simulink model "LQDG_Yaw"  (R2020a)
settings: Solver=ode3  StartTime=0.0  StopTime=10.0  FixedStep=0.01  RelTol=1e-3  EnableMultiTasking=on
undefined symbols (not defined in the file): weighting_matrix
libraries: arduinolib x5
settings Model: SILPILModeSetting=veronly  ExtModeTrigDuration=2  Creator=Ali  LastModifiedBy=Ali
settings OptimizationCC: EnhancedBackFolding=on  PassReuseOutputArgsAs=Individual arguments  ZeroExternalMemoryAtStartup=off  ZeroInternalMemoryAtStartup=off  MaxStackSize=64  OptimizeBlockOrder=speed  DifferentSizesBufferReuse=on  OptimizationCustomize=off  EfficientTunableParamExpr=on
settings DebuggingCC: ParameterTunabilityLossMsg=error
settings HardwareCC: ProdBitPerInt=16  ProdBitPerPointer=16  ProdBitPerSizeT=16  ProdBitPerPtrDiffT=16  ProdLargestAtomicFloat=None  ProdWordSize=8  ProdHWDeviceType=Atmel->AVR
settings SFSimCC: MATLABDynamicMemAlloc=off
settings RTWCC: SystemTargetFile=ert.tlc  HardwareBoard=Arduino Mega 2560  TLCOptions=-aInlineSetEventsForThisBaseRateFcn=TLC_FALSE -aSuppressMultiTaskScheduler=TLC_FALSE -aRateBasedStepFcn=1  TemplateMakefile=ert_default_tmf  Toolchain=Arduino AVR  BuildConfiguration=Faster Runs
settings CodeAppCC: ForceParamTrailComments=on  IgnoreCustomStorageClasses=off  OperatorAnnotations=on  SimulinkDataObjDesc=on  SFDataObjDesc=on  InsertBlockDesc=on
settings ERTTargetCC: SupportContinuousTime=on  SupportVariableSizeSignals=on  ExtModeStaticAllocSize=2048

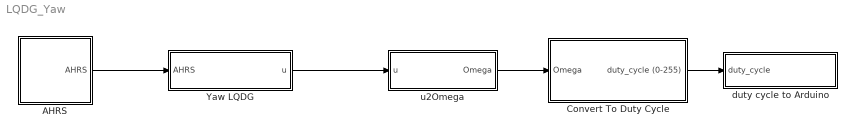
== system LQDG_Yaw ==
  " Yaw LQDG" : Subsystem
  AHRS : Subsystem
      mask Display: image('UM7.jpg'); % Use "Edit Image" on toolstrip to change.
  Convert To Duty Cycle : Subsystem
  duty cycle to Arduino : Subsystem
  u2Omega : Subsystem
  wires:
  u2Omega/1(Omega) -> Convert To Duty Cycle/1(Omega)
  AHRS/1(AHRS) -> " Yaw LQDG"/1(AHRS)
  " Yaw LQDG"/1(u) -> u2Omega/1(u)
  Convert To Duty Cycle/1(duty_cycle (0-255)) -> duty cycle to Arduino/1(duty_cycle)

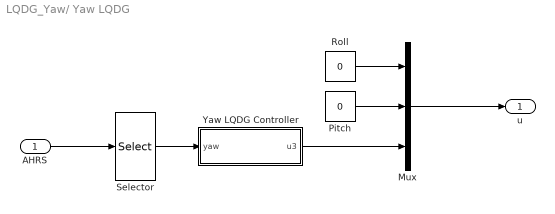
== system LQDG_Yaw/ Yaw LQDG ==
  AHRS : Inport
  Mux : Mux  Inputs=3
  Pitch : Constant  Value=0
  Roll : Constant  Value=0
  Selector : Selector  InputPortWidth=6  IndexOptions=Index vector (dialog)  Indices=[3 6]  OutputSizes=1
  Yaw LQDG Controller : Subsystem
  u : Outport
  wires:
  Mux/1 -> u/1
  AHRS/1 -> Selector/1
  Pitch/1 -> Mux/2
  Roll/1 -> Mux/1
  Selector/1 -> Yaw LQDG Controller/1(yaw)
  Yaw LQDG Controller/1(u3) -> Mux/3

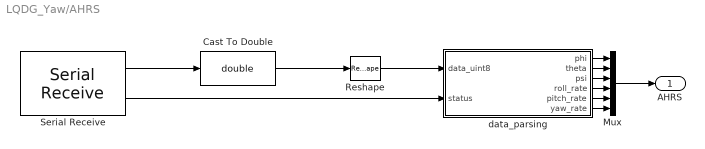
== system LQDG_Yaw/AHRS ==
  Cast To Double : DataTypeConversion  OutDataTypeStr=double
  Mux : Mux  Inputs=6
  Reshape : Reshape
  Serial Receive : arduinolib/Serial Receive  isARMArch=off  portNumber=1  DataType=uint8  Datalength=32  SampleTime=0.01  showOutStatus=on  blockPlatform=arduino
      settings: SourceProductBaseCode=ARDUINO
  data_parsing : MATLAB Function  TreatAsAtomicUnit=on
  AHRS : Outport
  wires:
  data_parsing/2(theta) -> Mux/2
  data_parsing/3(psi) -> Mux/3
  data_parsing/4(roll_rate) -> Mux/4
  Reshape/1 -> data_parsing/1(data_uint8)
  data_parsing/5(pitch_rate) -> Mux/5
  Serial Receive/2 -> data_parsing/2(status)
  data_parsing/6(yaw_rate) -> Mux/6
  Cast To Double/1 -> Reshape/1
  Serial Receive/1 -> Cast To Double/1
  data_parsing/1(phi) -> Mux/1
  Mux/1 -> AHRS/1

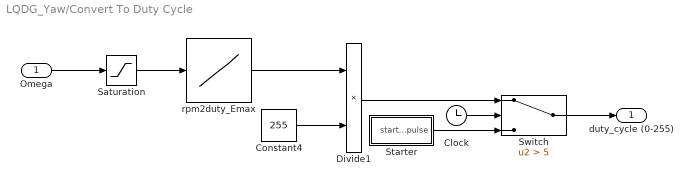
== system LQDG_Yaw/Convert To Duty Cycle ==
  Omega : Inport
  Clock : Clock
  Constant4 : Constant  Value=255
  Divide1 : Product  Inputs=**
  Saturation : Saturate  UpperLimit=6000  LowerLimit=1300
  Starter : Subsystem
  Switch : Switch  Criteria=u2 > Threshold  Threshold=5
  rpm2duty_Emax : Lookup_n-D  NumberOfTableDimensions=1  BreakpointsForDimension1=|  Table=|  RndMeth=Simplest  InputSameDT=on
      BreakpointsForDimension1=|
      | [1201
      | 2305
      | 3096
      | 3930
      | 4118
      | 4555
      | 5122
      | 5552
      | 5957
      | 6291
      | 6360]
      Table=|
      | [0.5
      | 0.55
      | 0.6
      | 0.65
      | 0.7
      | 0.75
      | 0.8
      | 0.85
      | 0.9
      | 0.95
      | 1]
  duty_cycle (0-255) : Outport
  wires:
  Switch/1 -> duty_cycle (0-255)/1
  Clock/1 -> Switch/2
  Divide1/1 -> Switch/1
  rpm2duty_Emax/1 -> Divide1/1
  Starter/1(start_pulse) -> Switch/3
  Omega/1 -> Saturation/1
  Constant4/1 -> Divide1/2
  Saturation/1 -> rpm2duty_Emax/1

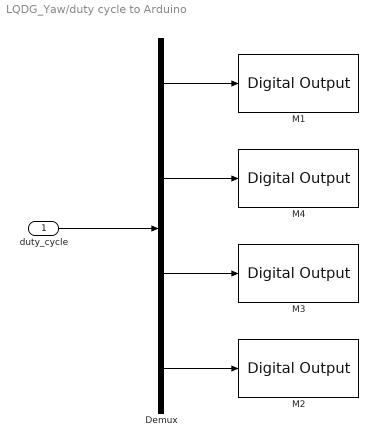
== system LQDG_Yaw/duty cycle to Arduino ==
  duty_cycle : Inport
  Demux : Demux
  M1 : arduinolib/Digital Output  pinNumber=8  Direction=output  blockPlatform=arduino
  M2 : arduinolib/Digital Output  pinNumber=9  Direction=output  blockPlatform=arduino
  M3 : arduinolib/Digital Output  pinNumber=10  Direction=output  blockPlatform=arduino
  M4 : arduinolib/Digital Output  pinNumber=11  Direction=output  blockPlatform=arduino
  wires:
  Demux/4 -> M2/1
  Demux/1 -> M1/1
  Demux/2 -> M4/1
  duty_cycle/1 -> Demux/1
  Demux/3 -> M3/1

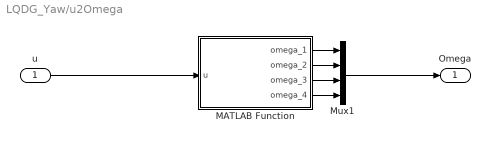
== system LQDG_Yaw/u2Omega ==
  u : Inport
  MATLAB Function : MATLAB Function  TreatAsAtomicUnit=on
  Mux1 : Mux
  Omega : Outport
  wires:
  Mux1/1 -> Omega/1
  MATLAB Function/2(omega_2) -> Mux1/2
  u/1 -> MATLAB Function/1(u)
  MATLAB Function/3(omega_3) -> Mux1/3
  MATLAB Function/1(omega_1) -> Mux1/1
  MATLAB Function/4(omega_4) -> Mux1/4

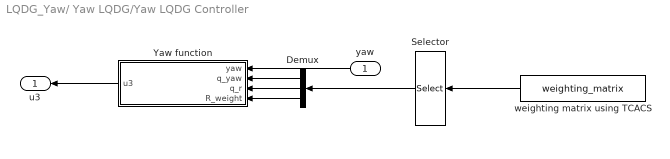
== system LQDG_Yaw/ Yaw LQDG/Yaw LQDG Controller ==
  yaw : Inport
  Demux : Demux  Outputs=3
  Selector : Selector  InputPortWidth=5  IndexOptions=Index vector (dialog)  Indices=[2 4 5]  OutputSizes=1
  Yaw function : MATLAB Function  TreatAsAtomicUnit=on
  weighting matrix using TCACS : Constant  Value=weighting_matrix
  u3 : Outport
  wires:
  Demux/2 -> Yaw function/3(q_r)
  Demux/1 -> Yaw function/2(q_yaw)
  Yaw function/1(u3) -> u3/1
  Demux/3 -> Yaw function/4(R_weight)
  yaw/1 -> Yaw function/1(yaw)
  weighting matrix using TCACS/1 -> Selector/1
  Selector/1 -> Demux/1

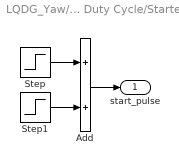
== system LQDG_Yaw/Convert To Duty Cycle/Starter ==
  Add : Sum
  Step : Step  After=140
  Step1 : Step  Time=2  After=-30
  start_pulse : Outport
  wires:
  Add/1 -> start_pulse/1
  Step/1 -> Add/1
  Step1/1 -> Add/2

== matlab function LQDG_Yaw/AHRS/data_parsing ==
  data: phi output size=1; data_uint8 input size=32; theta output size=1; psi output size=1; roll_rate output size=1; pitch_rate output size=1; yaw_rate output size=1; status input
function [phi,theta,psi,roll_rate,pitch_rate,yaw_rate] = fcn(data_uint8, status)
persistent stepp check_sum...
    phi_p theta_p psi_p roll_rate_p pitch_rate_p yaw_rate_p...
    phi_last theta_last psi_last roll_rate_last pitch_rate_last yaw_rate_last;
%% Initialize
if isempty(stepp)
    stepp=0;
    check_sum=0;
    phi_p=0;
    theta_p=0;
    psi_p=0;
    roll_rate_p=0;
    pitch_rate_p=0;
    yaw_rate_p=0;
    phi_last=0;
    theta_last=0;
    psi_last=0;
    roll_rate_last=0;
    pitch_rate_last=0;
    yaw_rate_last=0;
end
angle_scale=.0109863;  % 1/91.0222
rate_scale=1/16;
%% Check Each Byte
if status
    for i = 1:length(data_uint8)
        if (data_uint8(i)==115 && stepp==0)
            stepp=1;
            check_sum=data_uint8(i);
        elseif(stepp==1 && data_uint8(i)==110)
            stepp=stepp+1;
            check_sum=check_sum+data_uint8(i);
        elseif(stepp==2 && data_uint8(i)==112)
            stepp=stepp+1;
            check_sum=check_sum+data_uint8(i);
        elseif(stepp==3 && data_uint8(i)==212)
            stepp=stepp+1;
            check_sum=check_sum+data_uint8(i);
        elseif(stepp==4 && data_uint8(i)==112)
            stepp=stepp+1;
            check_sum=check_sum+data_uint8(i);
        elseif(stepp==5)
            phi_p=data_uint8(i)*256;
            stepp=stepp+1;
            check_sum=check_sum+data_uint8(i);
        elseif(stepp==6)
            phi_p=phi_p+data_uint8(i);
            stepp=stepp+1;
            check_sum=check_sum+data_uint8(i);
        elseif(stepp==7)
            theta_p=data_uint8(i)*256;
            stepp=stepp+1;
            check_sum=check_sum+data_uint8(i);
        elseif(stepp==8)
            theta_p=theta_p+data_uint8(i);
            stepp=stepp+1;
            check_sum=check_sum+data_uint8(i);
        elseif(stepp==9)
            psi_p=data_uint8(i)*256;
            stepp=stepp+1;
            check_sum=check_sum+data_uint8(i);
        elseif(stepp==10)
            psi_p=psi_p+data_uint8(i);
            stepp=stepp+1;
            check_sum=check_sum+data_uint8(i);
        elseif(stepp==11 || stepp==12)
            if(data_uint8(i)==0)
                stepp=stepp+1;
            else
                stepp=0;
            end
        elseif(stepp==13)
            roll_rate_p=data_uint8(i)*256;
            stepp=stepp+1;
            check_sum=check_sum+data_uint8(i);
        elseif(stepp==14)
            roll_rate_p=roll_rate_p+data_uint8(i);
            stepp=stepp+1;
            check_sum=check_sum+data_uint8(i);
        elseif(stepp==15)
            pitch_rate_p=data_uint8(i)*256;
            stepp=stepp+1;
            check_sum=check_sum+data_uint8(i);
        elseif(stepp==16)
            pitch_rate_p=pitch_rate_p+data_uint8(i);
            stepp=stepp+1;
            check_sum=check_sum+data_uint8(i);
        elseif(stepp==17)
            yaw_rate_p=data_uint8(i)*256;
            stepp=stepp+1;
            check_sum=check_sum+data_uint8(i);
        elseif(stepp==18)
            yaw_rate_p=yaw_rate_p+data_uint8(i);
            stepp=stepp+1;
            check_sum=check_sum+data_uint8(i);
        elseif(stepp==19 || stepp==20)
            if(data_uint8(i)==0)
                stepp=stepp+1;
            else
                stepp=0;
            end
        elseif(stepp==21 || stepp==22 || stepp==23 || stepp==24)
            stepp=stepp+1;
            check_sum=check_sum+data_uint8(i);
        elseif(stepp==25)
            if (floor(check_sum/256)==data_uint8(i))
                stepp=stepp+1;
            else
                stepp=0;
            end
        elseif(stepp==26)
            if(mod(check_sum,256)==data_uint8(i))
                phi_last=double(typecast(uint16(phi_p), 'int16'))*angle_scale;
                if mod(phi_last,360)>180
                    phi_last=mod(phi_last,360)-360;
                else
                    phi_last=mod(phi_last,360);
                end
                theta_last=double(typecast(uint16(theta_p), 'int16'))*angle_scale;
                if mod(theta_last,360)>180
                    theta_last=mod(theta_last,360)-360;
                else
                    theta_last=mod(theta_last,360);
                end
                psi_last=double(typecast(uint16(psi_p), 'int16'))*angle_scale;
                if mod(psi_last,360)>180
                    psi_last=mod(psi_last,360)-360;
                else
                    psi_last=mod(psi_last,360);
                end
                roll_rate_last=double(typecast(uint16(roll_rate_p), 'int16'))*rate_scale;
                if mod(roll_rate_last,360)>180
                    roll_rate_last=mod(roll_rate_last,360)-360;
                else
                    roll_rate_last=mod(roll_rate_last,360);
                end
                pitch_rate_last=double(typecast(uint16(pitch_rate_p), 'int16'))*rate_scale;
                if mod(pitch_rate_last,360)>180
                    pitch_rate_last=mod(pitch_rate_last,360)-360;
                else
                    pitch_rate_last=mod(pitch_rate_last,360);
                end
                yaw_rate_last=double(typecast(uint16(yaw_rate_p), 'int16'))*rate_scale;
                if mod(yaw_rate_last,360)>180
                    yaw_rate_last=mod(yaw_rate_last,360)-360;
                else
                    yaw_rate_last=mod(yaw_rate_last,360);
                end
            end
            stepp=0;
        end
    end
end

%% Assign Last True Data to Output
phi=phi_last;
theta=theta_last;
psi=psi_last;
roll_rate=roll_rate_last;
pitch_rate=pitch_rate_last;
yaw_rate=yaw_rate_last;

== matlab function LQDG_Yaw/ Yaw LQDG/Yaw LQDG Controller/Yaw function ==
  data: yaw input; u3 output; q_yaw input; q_r input; R_weight input
function u3 = fcn(yaw, q_yaw, q_r, R_weight)
% QuadConstants;
%%% constans %%%
% Distance between rotor center to quad center (m)
% d_cg = 0.295;
% Distance between D point to quad center (m)
% h_cg = 0.0078;
% Thrust factor (non dimensional)
% b = 1.10794e-5;
% Rotor torque drag factor (non dimensional)
d = 3.2e-6;
% Total mass (kg)
% m_tot = 1.774;
% Quad Moment of inertia respect to axix X Body (kg.m^2)
% J_xx = 0.0297598;
% Quad Moment of inertia respect to axix Y Body (kg.m^2)
% J_yy = 0.0298565;
% Quad Moment of inertia respect to axix Y Body (kg.m^2)
J_zz = 0.058510;
% Quad blade Moment (kg.m^2)
% J_R = 4.439e-5;
% Mass on X axis bearing (kg)
% m1 = 1.272;
% Mass on Y axis bearing (kg)
% m2 = 1.074;
% Mass on Z axis bearing (kg)
% m3 = 1.693;
% Bearing radius in X axix (m)
% r_x = 0.01;
% Bearing radius in Y axix (m)
% r_y = 0.01;
% Bearing radius in Z axix (m)
% r_z = 0.025;
% Static bearing friction (non dimensional)
% miu_s = 0.003;
% Dynamic bearing friction (non dimensional)
% miu_k = 0.002;
% Motor constant (non dimensional)
% tau = 0.15;
% Delay of motor (sec)
% T_d = 0.02;
% Gravity force (m/s^2)
% g = 9.81;
% A Constants
% A1 = (h_cg * g * m_tot) / (m_tot * h_cg^2 + J_xx);
% A2 = (2*m_tot * h_cg^2 + J_yy -J_zz) / (m_tot * h_cg^2 + J_xx);
% A3 = (b * d_cg) / (m_tot * h_cg^2 + J_xx);
% A4 = (J_R) / (m_tot * h_cg^2 + J_xx);
% A5 = (m1 * g * miu_k * r_x) / (m_tot * h_cg^2 + J_xx);
% B Constants
% B1 = (h_cg * g * m_tot) / (m_tot * h_cg^2 + J_yy);
% B2 = (-2*m_tot * h_cg^2 - J_xx + J_zz) / (m_tot * h_cg^2 + J_yy);
% B3 = (b * d_cg) / (m_tot * h_cg^2 + J_yy);
% B4 = (-J_R) / (m_tot * h_cg^2 + J_yy);
% B5 = (m2 * g * miu_k * r_y) / (m_tot * h_cg^2 + J_yy);
% C Constants
% C1 = (J_xx - J_yy) / (J_zz);
C2 = (d) / (J_zz);
% C3 = (m3 * g * miu_k * r_z) / (J_zz);
% omega for linearzation 2000 RPM
% Omega = 2000 / 60 * 2 * pi;

A33    = 0; %da3dx3
A36    = 1; %da3dx6
A63    = 0; %da6dx3
A66    = 0; %da6dx6


A      = [A33, A36 ;
          A63, A66];
B      = [0  ;
          C2];
a      = A(2);
b      = B(2);

q1     = 10^q_yaw;
q2     = 10^q_r;
R1     = 1;
R2     = 10^R_weight;
R1_inv = R1^-1;
R2_inv = R2^-1;
k1_ans = zeros(2, 2);
k2_ans = zeros(2, 2);

% algebraic_riccati = K * A + A' * K - K * B * R^-1 * B' * K + Q;
% first equation q1 + 2*a*k12 - (b^2*k12^2)/R = 0
% Ans1 K12 = -m*(k + (k^2 + Q11)^(1/2))
% Ans2 K12 = -m*(k - (k^2 + Q11)^(1/2))
valid_ans = false; % answer validation for statble system
k12_1 = zeros(1, 2);
k12_2 = zeros(1, 2);
k12_1(1) =   (R1*R2*a + R1*b^2*((R1*R2*(R1*R2*a^2 + R1*b^2*q1 + R2*b^2*q1))/(b^4*(R1 + R2)^2))^(1/2) + R2*b^2*((R1*R2*(R1*R2*a^2 + R1*b^2*q1 + R2*b^2*q1))/(b^4*(R1 + R2)^2))^(1/2))/(R1*b^2 + R2*b^2);
k12_1(2) =  -(R1*b^2*((R1*R2*(R1*R2*a^2 + R1*b^2*q1 + R2*b^2*q1))/(b^4*(R1 + R2)^2))^(1/2) - R1*R2*a + R2*b^2*((R1*R2*(R1*R2*a^2 + R1*b^2*q1 + R2*b^2*q1))/(b^4*(R1 + R2)^2))^(1/2))/(R1*b^2 + R2*b^2);
k12_2(1) =  (R1*R2*a + R1*b^2*((R1*R2*(R1*R2*a^2 + R1*b^2*q1 + R2*b^2*q1))/(b^4*(R1 + R2)^2))^(1/2) + R2*b^2*((R1*R2*(R1*R2*a^2 + R1*b^2*q1 + R2*b^2*q1))/(b^4*(R1 + R2)^2))^(1/2))/(R1*b^2 + R2*b^2);
for i = 1:length(k12_1)
    % Second equation 
    % 1 (b^2*k22_1^2)/R1 + (k22_2*b^2*k22_1)/R2 - 2*k12_1 - q2 = 0
    % 2 (b^2*k22_2^2)/R2 + (k22_1*b^2*k22_2)/R1 - 2*k12_2 - q2
    % Ans1 K22_1 =  -((2*k12_1 + q2)*((R1*R2*
    % (2*k12_2 + q2)^2)/(b^2*(2*R1*k12_2 + 2*R2*k12_1 + R1*q2 + R2*q2)))
    % ^(1/2))/(2*k12_2 + q2)
    
    % Ans2 K22_1 = ((2*k12_1 + q2)*((R1*R2*(2*k12_2 + q2)^2)
    % /(b^2*(2*R1*k12_2 + 2*R2*k12_1 + R1*q2 + R2*q2)))^(1/2))/(2*k12_2 + q2)
    
    % Ans1 K22_2 =  -((R1*R2*(2*k12_2 + q2)^2)/(b^2*
    % (2*R1*k12_2 + 2*R2*k12_1 + R1*q2 + R2*q2)))^(1/2)

    % Ans1 K22_2 = ((R1*R2*(2*k12_2 + q2)^2)/
    % (b^2*(2*R1*k12_2 + 2*R2*k12_1 + R1*q2 + R2*q2)))^(1/2)
    
    k22_1 = zeros(1, 2);
    k22_2 = zeros(1, 2);
    valid22 = [true; true]; % for validation in complex number
    if ((R1*R2*(2*k12_2(i) + q2)^2)/(b^2*(2*R1*k12_2(i) + 2*R2*k12_1(i) + R1*q2 + R2*q2))) < 0 
        valid22(i) = false;
    else
        k22_1(1) = -((2*k12_1(i) + q2)*((R1*R2*(2*k12_2(i) + q2)^2)/(b^2*(2*R1*k12_2(i) + 2*R2*k12_1(i) + R1*q2 + R2*q2)))^(1/2))/(2*k12_2(i) + q2);
    end
    if ((R1*R2*(2*k12_2(i) + q2)^2)/(b^2*(2*R1*k12_2(i) + 2*R2*k12_1(i) + R1*q2 + R2*q2))) < 0
        valid22(i) = false;
    else
        k22_1(2) =  ((2*k12_1(i) + q2)*((R1*R2*(2*k12_2(i) + q2)^2)/(b^2*(2*R1*k12_2(i) + 2*R2*k12_1(i) + R1*q2 + R2*q2)))^(1/2))/(2*k12_2(i) + q2);
    end
    if ((R1*R2*(2*k12_2(i) + q2)^2)/(b^2*(2*R1*k12_2(i) + 2*R2*k12_1(i) + R1*q2 + R2*q2))) < 0
        valid22(i) = false;
    else
        k22_2(1) = -((R1*R2*(2*k12_2(i) + q2)^2)/(b^2*(2*R1*k12_2(i) + 2*R2*k12_1(i) + R1*q2 + R2*q2)))^(1/2);
        k22_2(2) =  ((R1*R2*(2*k12_2(i) + q2)^2)/(b^2*(2*R1*k12_2(i) + 2*R2*k12_1(i) + R1*q2 + R2*q2)))^(1/2);
    end
    for j = 1:length(k22_1)
        if valid22(i) == false
            continue
        end
        % Last equation 
        % 1 (b^2*k12_1*k22_1)/R1 - a*k22_1 - k11_1 + (b^2*k12_2*k22_1)/R2
        % Ans k11_1 = (b^2*k12_1*k22_1)/R1 - a*k22_1 + (b^2*k12_2*k22_1)/R2
        % Ans k11_2 = (b^2*k12_1*k22_1)/R1 - a*k22_1 + (b^2*k12_2*k22_1)/R2
        k11_1 = (b^2*k12_1(i)*k22_1(j))/R1 - a*k22_1(j) + (b^2*k12_2(i)*k22_1(j))/R2;
        k11_2 = (b^2*k12_1(i)*k22_2(j))/R1 - a*k22_2(j) + (b^2*k12_2(i)*k22_2(j))/R2;
        temp_K_1 = zeros(2, 2);
        temp_K_1(1, 1) = k11_1;
        temp_K_1(1, 2) = k12_1(i);
        temp_K_1(2, 1) = k12_1(i);
        temp_K_1(2, 2) = k22_1(j);
        temp_K_2 = zeros(2, 2);
        temp_K_2(1, 1) = k11_2;
        temp_K_2(1, 2) = k12_2(i);
        temp_K_2(2, 1) = k12_2(i);
        temp_K_2(2, 2) = k22_2(j);
        if all(eig(A + (-B*R1_inv*B'*temp_K_1 - B*R2_inv*B'*temp_K_2)) < 0)
            k1_ans = temp_K_1;
            k2_ans = temp_K_2;
            valid_ans = true;
            break;
        end
        if valid_ans == true
            break;
        end
    end
    if valid_ans == true
        break;
    end
end

u3 = (-R1_inv*B'*k1_ans -R2_inv*B'*k2_ans) *yaw;

== matlab function LQDG_Yaw/u2Omega/MATLAB Function ==
  data: u input; omega_1 output; omega_2 output; omega_3 output; omega_4 output
function [omega_1, omega_2, omega_3, omega_4] = fcn(u)
u1 = u(1);
u2 = u(2);
u3 = u(3);
% control effort
u4 = ones(1, length(u1)) * 4 * rpm2rad_sec(3000)^2;
% calculate omega
omega_1 = sqrt((u4 + u3 + 2 * u2) / 4);
omega_3 = sqrt((u4 + u3 - 2 * u2) / 4);
omega_2 = sqrt((u4 - u3 + 2 * u1) / 4);
omega_4 = sqrt((u4 - u3 - 2 * u1) / 4);
end
%% functions
% rpm to rad/sec
function rad = rpm2rad_sec(rpm)
rad = rpm / 60 * 2 * pi;
end
